simulink model "robot"  (R2024b)
settings: Solver=VariableStepAuto  StartTime=0.0  StopTime=Tf  RelTol=1e-3
values from neighbouring files (symbols this model uses):
  param = [Km Tau R]    [simple_motor_traject.m]
  pre_gain_v = 1/0.8    (= 1.25)    [simple_motor_traject.m]
  pre_gain_w = 1/0.9    (= 1.11111111111)    [simple_motor_traject.m]
  px0 = 0    [simple_motor_traject.m]
  py0 = 0    [simple_motor_traject.m]
  Tf = 100    [simple_motor_traject.m]
  u_sat = 0.5*V_max    (= 0.35)    [simple_motor_traject.m]
  x_ref = 10    [simple_motor_traject.m]
  y_ref = 15    [simple_motor_traject.m]
settings Model: Creator=gabri  LastModifiedBy=gabri
settings RTWCC: GPUComputeCapability=3.5

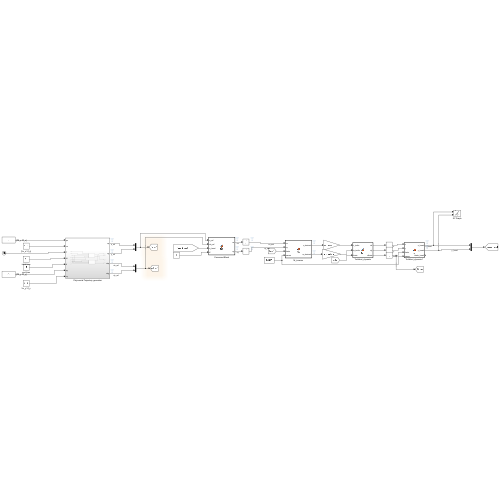
[thumbnail: Simulink's stored preview of the top-level diagram]
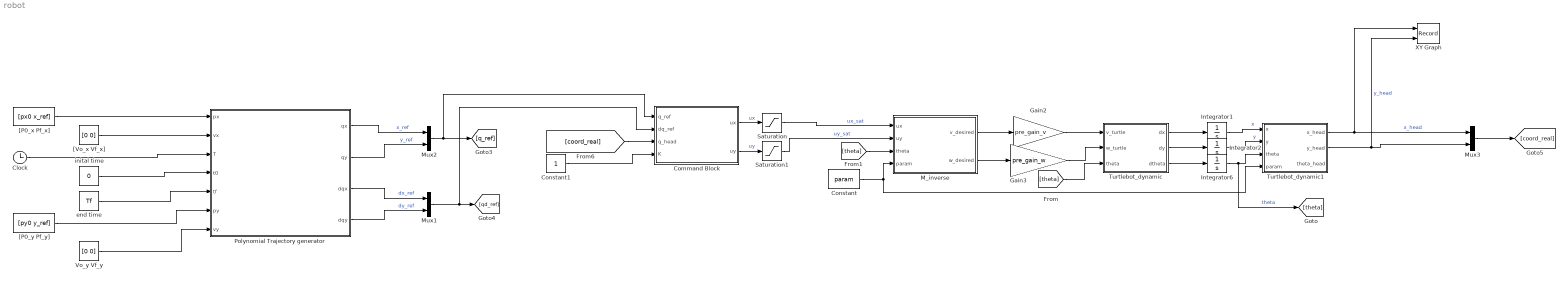
== system robot ==
  Clock : Clock
  Command Block : MATLAB Function  TreatAsAtomicUnit=on
  Constant : Constant  Value=param
  Constant1 : Constant
  Gain2 : Gain  Gain=pre_gain_v
  Gain3 : Gain  Gain=pre_gain_w
  Integrator1 : Integrator  InitialCondition=px0
  Integrator2 : Integrator  InitialCondition=px0
  Integrator6 : Integrator  InitialCondition=px0
  M_inverse : MATLAB Function  TreatAsAtomicUnit=on
  Mux1 : Mux  Inputs=2
  Mux2 : Mux  Inputs=2
  Mux3 : Mux  Inputs=2
  Polynomial Trajectory generator : Subsystem
  Saturation : Saturate  UpperLimit=u_sat  LowerLimit=-u_sat
  Saturation1 : Saturate
  Turtlebot_dynamic : MATLAB Function  TreatAsAtomicUnit=on
  Turtlebot_dynamic1 : MATLAB Function  TreatAsAtomicUnit=on
  Vo_y Vf_y : Constant  Value=[0 0]
  XY Graph : Record  FileSettingsInternal="{\"entries\":[{\"content\":{\"excelSettings\":{\"content\":{},\"type\":\"Streamout.ExcelSettings\"}},\"type\":\"Streamout.FileSettingStorage\",\"uuid\":\"\"}],\"packageUris\":[\"http:\\/\\/schema.mathworks.com\\/mf0\\/streamout_blocks\\/R2020a\"],\"version\":\"1.0\"}"  Layout=[1 1]  SignalsInternal="{\"entries\":[{\"content\":{\"signals\":[{\"content\":{\"blockPath\":[],\"dimensions\":[1],\"domain\":\"\",\"lineColor\":\"#a2142f\",\"plots\":[ 1 ],\"port\":1,\"sid\":[\"\"],\"signalID\":1,\"signalName\":\"x_head\"},\"type\":\"RecordBlkView.Signal\",\"uuid\":\"\"},{\"content\":{\"blockPath\":[],\"dimensions\":[1],\"domain\":\"\",\"lineColor\":\"#139fff\",\"plots\":[ 1 ],\"port\":2,\"sid\":[\"\"],\"signalID\":2,\"signalName\":\"y_head\"},\"type\":\"RecordBlkView.Signal\",\"uuid\":\"\"}]},\"type\":\"RecordBlkView.InputSignals\",\"uuid\":\"\"}],\"packageUris\":[\"http:\\/\\/schema.mathworks.com\\/mf0\\/streamout_blocks\\/R2020a\"],\"version\":\"1.0\"}"  VisualizationBindings="{\"xyplotplugin\":{\"info\":[{\"series\":[{\"bindingParametersList\":[{\"parameter\":\"X-Axis\",\"signalID\":1,\"signalName\":\"x_head\"},{\"parameter\":\"Y-Axis\",\"signalID\":2,\"signalName\":\"y_head\"}],\"seriesID\":0}],\"subplotID\":1}]}}"  CompatibilityTag=XY
  "[P0_x Pf_x]" : Constant  Value=[px0 x_ref]
  "[P0_y Pf_y]" : Constant  Value=[py0 y_ref]
  "[Vo_x Vf_x]" : Constant  Value=[0 0]
  end time : Constant  Value=Tf
  inital time : Constant  Value=0
  wires:
  "[P0_x Pf_x]"/1 -> Polynomial Trajectory generator/1(px)
  "[Vo_x Vf_x]"/1 -> Polynomial Trajectory generator/2(vx)
  Clock/1 -> Polynomial Trajectory generator/3(T)
  inital time/1 -> Polynomial Trajectory generator/4(t0)
  end time/1 -> Polynomial Trajectory generator/5(tf)
  "[P0_y Pf_y]"/1 -> Polynomial Trajectory generator/6(py)
  Vo_y Vf_y/1 -> Polynomial Trajectory generator/7(vy)
  Polynomial Trajectory generator/1(qx) -> Mux2/1  "x_ref"
  Polynomial Trajectory generator/2(qy) -> Mux2/2  "y_ref"
  Polynomial Trajectory generator/4(dqy) -> Mux1/2  "dy_ref"
  Polynomial Trajectory generator/3(dqx) -> Mux1/1  "dx_ref"
  Mux2/1 -> Command Block/1(q_ref), [q_ref]
  Mux1/1 -> Command Block/2(dq_ref), [qd_ref]
  Command Block/1(ux) -> Saturation/1  "ux"
  Command Block/2(uy) -> Saturation1/1  "uy"
  [coord_real] -> Command Block/3(q_head)
  Constant1/1 -> Command Block/4(K)
  M_inverse/1(v_desired) -> Gain2/1
  M_inverse/2(w_desired) -> Gain3/1
  Turtlebot_dynamic/1(dx) -> Integrator1/1
  Turtlebot_dynamic/2(dy) -> Integrator2/1
  Turtlebot_dynamic/3(dtheta) -> Integrator6/1
  Integrator1/1 -> Turtlebot_dynamic1/1(x)  "x"
  Integrator2/1 -> Turtlebot_dynamic1/2(y)  "y"
  Integrator6/1 -> [theta], Turtlebot_dynamic1/3(theta)  "theta"
  Mux3/1 -> [coord_real]
  Turtlebot_dynamic1/1(x_head) -> XY Graph/1, Mux3/1  "x_head"
  Turtlebot_dynamic1/2(y_head) -> XY Graph/2, Mux3/2  "y_head"
  Constant/1 -> Turtlebot_dynamic1/4(param), M_inverse/4(param)
  [theta] -> Turtlebot_dynamic/3(theta)
  [theta] -> M_inverse/3(theta)
  Gain2/1 -> Turtlebot_dynamic/1(v_turtle)
  Gain3/1 -> Turtlebot_dynamic/2(w_turtle)
  Saturation/1 -> M_inverse/1(ux)  "ux_sat"
  Saturation1/1 -> M_inverse/2(uy)  "uy_sat"

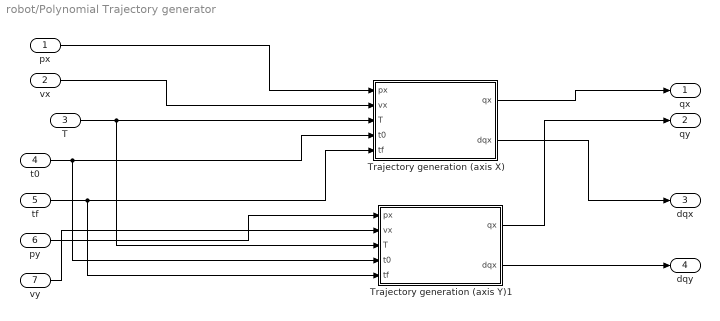
== system robot/Polynomial Trajectory generator ==
  px : Inport
  vx : Inport  Port=2
  T : Inport  Port=3
  t0 : Inport  Port=4
  tf : Inport  Port=5
  py : Inport  Port=6
  vy : Inport  Port=7
  Trajectory generation (axis X) : MATLAB Function  TreatAsAtomicUnit=on
  Trajectory generation (axis Y)1 : MATLAB Function  TreatAsAtomicUnit=on
  qx : Outport
  qy : Outport  Port=2
  dqx : Outport  Port=3
  dqy : Outport  Port=4
  wires:
  Trajectory generation (axis X)/2(dqx) -> dqx/1
  T/1 -> Trajectory generation (axis Y)1/3(T), Trajectory generation (axis X)/3(T)
  vx/1 -> Trajectory generation (axis X)/2(vx)
  tf/1 -> Trajectory generation (axis Y)1/5(tf), Trajectory generation (axis X)/5(tf)
  t0/1 -> Trajectory generation (axis Y)1/4(t0), Trajectory generation (axis X)/4(t0)
  Trajectory generation (axis X)/1(qx) -> qx/1
  Trajectory generation (axis Y)1/2(dqx) -> dqy/1
  Trajectory generation (axis Y)1/1(qx) -> qy/1
  px/1 -> Trajectory generation (axis X)/1(px)
  py/1 -> Trajectory generation (axis Y)1/1(px)
  vy/1 -> Trajectory generation (axis Y)1/2(vx)

== matlab function robot/M_inverse ==
  data: ux input; v_desired output; uy input; theta input; param input; w_desired output
function [v_desired,w_desired] = fcn(ux, uy, theta, param)

R = param(3);

M_inv = [cos(theta), sin(theta);
    (-1/R)*sin(theta), (1/R)*cos(theta)];

v_desired = M_inv(1,1)* ux + M_inv(1,2)*uy;
w_desired = M_inv(2,1)* ux + M_inv(2,2)*uy;

== matlab function robot/Polynomial Trajectory generator/Trajectory generation (axis X) ==
  data: px input; qx output; vx input; T input; t0 input; tf input; dqx output
function [qx,dqx] = fcn(px,vx,T,t0,tf)

p0 = px(1);
pf = px(2);

v0 = vx(1);
vf = vx(2);

a0 = p0;
a1 = v0*(tf-t0);
a3 = ((vf-v0)*(tf-t0))-(2*(pf-p0)-(2*v0*(tf-t0)));
a2 = (pf-p0)-v0*(tf-t0)-a3;

lambda_t = (T-t0)/(tf-t0);

if(T<tf)
    qx = a0 + a1*lambda_t + a2*lambda_t^2 + a3*lambda_t^3;
    dqx = (a1 + 2*a2*lambda_t + 3*a3*lambda_t^2)/(tf-t0);    
else
    qx = pf;
    dqx = vf;
end

== matlab function robot/Polynomial Trajectory generator/Trajectory generation (axis Y)1 ==
  data: px input; qx output; vx input; T input; t0 input; tf input; dqx output
function [qx,dqx] = fcn(px,vx,T,t0,tf)

p0 = px(1);
pf = px(2);

v0 = vx(1);
vf = vx(2);

a0 = p0;
a1 = v0*(tf-t0);
a3 = ((vf-v0)*(tf-t0))-(2*(pf-p0)-(2*v0*(tf-t0)));
a2 = (pf-p0)-v0*(tf-t0)-a3;

lambda_t = (T-t0)/(tf-t0);

if(T<tf)
    qx = a0 + a1*lambda_t + a2*lambda_t^2 + a3*lambda_t^3;
    dqx = (a1 + 2*a2*lambda_t + 3*a3*lambda_t^2)/(tf-t0);    
else
    qx = pf;
    dqx = vf;
end

== matlab function robot/Command Block ==
  data: q_ref input; ux output; dq_ref input; q_head input; K input; uy output
function [ux,uy] = fcn(q_ref,dq_ref,q_head,K)

x_ref = q_ref(1);
y_ref = q_ref(2);

dx_ref = dq_ref(1);
dy_ref = dq_ref(2);

x_head = q_head(1);
y_head = q_head(2);

ux = K*(x_ref - x_head);
uy = K*(y_ref - y_head);

== matlab function robot/Turtlebot_dynamic ==
  data: v_turtle input; dx output; w_turtle input; dy output; theta input; dtheta output
function [dx, dy, dtheta] = fcn(v_turtle, w_turtle, theta)

dx = cos(theta)*v_turtle*0.8;
dy = sin(theta)*v_turtle*0.8;
dtheta = w_turtle*0.9;

== matlab function robot/Turtlebot_dynamic1 ==
  data: x_head output; x input; y input; y_head output; theta input; theta_head output; param input
function [x_head, y_head, theta_head] = fcn(x,y,theta,param)

R = param(3);

x_head = x + R*cos(theta);
y_head = y + R*sin(theta);
theta_head = theta;
